simulink model "radio"  (R2023a)
settings: Solver=VariableStepAuto  StartTime=0.0  StopTime=10.0  RelTol=1e-3
libraries: dspvision x2, simulink x1, commanabbnd3 x1, zedboardfmc234_lib x1
settings Model: Creator=Lenovo  LastModifiedBy=Lenovo

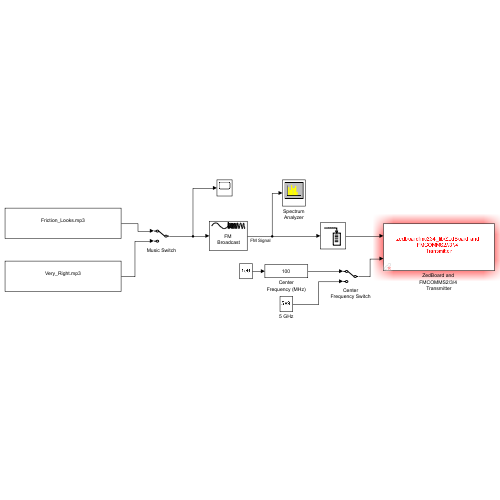
[thumbnail: Simulink's stored preview of the top-level diagram]
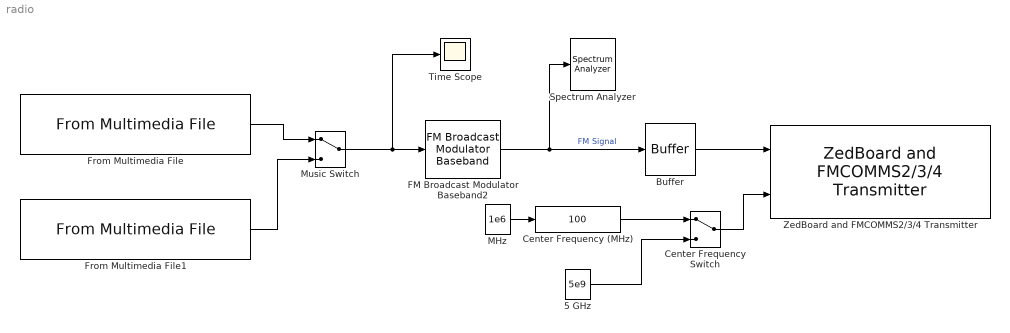
== system radio ==
  5 GHz : Constant  Value=5e9  VectorParams1D=off  SampleTime=192000/960000  FramePeriod=-1
  Buffer : Buffer  N=192000  OutputFrames=off
  Center Frequency (MHz) : simulink/Math Operations/Slider Gain  gain=100  low=98  high=102
  Center Frequency Switch : ManualSwitch
  FM Broadcast Modulator Baseband2 : commanabbnd3/FM Broadcast Modulator Baseband  SampleRate=960000  FrequencyDeviation=75000  FilterTimeConstant=7.5e-5  AudioSampleRate=48000  Stereo=on  RBDS=off  RBDSSamplesPerSymbol=10  SimulateUsing=Code generation
  From Multimedia File : dspvision/From Multimedia File  inputFilename=D:\LO_SHIH_AN\SDR\Matlab_object\SDR_FM_Radio\no_copyright_music\Friction_Looks.mp3  readRange=[1 Inf]  loop=on  numPlays=10  outputStreams=Audio only  videoDataType=single  audioDataType=double  inheritSampleTime=on  userDefinedSampleTime=1/4410  noAudioOutput=off  isIntensityVideo=off  fourcc=RGB  colorVideoFormat=Separate color signals  outputEOF=off  dataOrg=Column-major  audioFrameSize=48000  computeAudioFrameSize=off  outSamplingMode=Sample based
  From Multimedia File1 : dspvision/From Multimedia File  inputFilename=D:\LO_SHIH_AN\SDR\Matlab_object\SDR_FM_Radio\no_copyright_music\Very_Right.mp3  readRange=[1 Inf]  loop=on  numPlays=10  outputStreams=Audio only  videoDataType=single  audioDataType=double  inheritSampleTime=on  userDefinedSampleTime=1/4800  noAudioOutput=off  isIntensityVideo=off  fourcc=RGB  colorVideoFormat=Separate color signals  outputEOF=off  dataOrg=Column-major  audioFrameSize=48000  computeAudioFrameSize=off  outSamplingMode=Sample based
  MHz : Constant  Value=1e6  VectorParams1D=off  SampleTime=192000/960000  FramePeriod=-1
  Music Switch : ManualSwitch
  Spectrum Analyzer : SpectrumAnalyzer  WindowPosition=[1212 180 483 666]  ScopeFrameLocation=window  ViewType=Spectrum and spectrogram  Method=Welch  SampleRate=960000  Span=27930  StartFrequency=-13965  StopFrequency=13965  AveragingMethod=Running  YLimits=[-159.00256673081184999,35.803452450867595758]  ColorLimits=[-90.984095857497905513,17.091530854464384248]  ShowLegend=on  DefaultConfigurationName=spbscopes.SpectrumAnalyzerBlockCfg
  Time Scope : Scope
  ZedBoard and FMCOMMS2/3/4 Transmitter : zedboardfmc234_lib/ZedBoard and  FMCOMMS2//3//4  Transmitter  IPAddress=192.168.3.2  CenterFrequencySource=Input port  CenterFrequency=2400000000  GainSource=Dialog  Gain=0  ChannelMapping=1  BasebandSampleRate=960000  EnableBurstMode=off  NumFramesInBurst=20  DMATimeoutValue=1  EnableTxPrimingMode=on  blockMode=Normal  LostSamplesOutputPort=off  OverflowOutputPort=off  SimulateUsing=Code generation  DataSourceSelect=Host  DDSFrequency=[ 1000000, 1000000; 1000000, 1000000 ]  DDSPhase=[ 0, 0; 0, 0 ]  DDSScale=[ 250000, 250000; 250000, 250000 ]  BypassUserLogic=off  ShowAdvancedProperties=on  ShowInternalProperties=off  subDeviceList=zynqTransmitter  sdrExecutionMode=HW  dataUDPPort=-1  ctrlUDPPort=-1  FIRCoefficientSize=[ 128; 128 ]  FIRCoefficients=[ 111, -87, 147, -127, -18, -286, -312, -555, -601, -722, -642, -555, -303, -66, 221, 393, 488, 403, 219, -74, -343, -550, -582, -450, -146, 221, 569, 759, 735, 463, 20, -487, -885, -1048, -883, -418, 243, 897, 1340, 1394, 1002, 228, -715, -1549, -1980, -1819, -1028, 217, 1583, 2635, 2980, 2377, 853, -1275, -3435, -4926, -5080, -3454, 40, 5065, 10903, 16581, 21085, 23573, 23573, 21085, 16581, 10903, 5065, 40, -3454, -5080, -4926, -3435, -1275, 853, 2377, 2980, 2635, 1583, 217, -1028, -1819, -1980, -1549, -715, 228, 1002, 1394, 1340, 897, 243, -418, -883, -1048, -885, -487, 20, 463, 735, 759, 569, 221, -146, -450, -582, -550, -343, -74, 219, 403, 488, 393, 221, -66, -303, -555, -642, -722, -601, -555, -312, -286, -18, -127, 147, -87, 111; 382, -200, 711, -41, 645, 36, 346, -194, -119, -543, -472, -646, -404, -312, 45, 197, 413, 346, 241, -93, -373, -680, -755, -689, -356, 51, 515, 795, 870, 609, 136, -488, -1009, -1303, -1191, -712, 69, 885, 1516, 1692, 1336, 468, -662, -1740, -2378, -2329, -1494, -55, 1620, 2995, 3584, 3045, 1368, -1121, -3755, -5708, -6156, -4542, -710, 4969, 11669, 18243, 23486, 26391, 26391, 23486, 18243, 11669, 4969, -710, -4542, -6156, -5708, -3755, -1121, 1368, 3045, 3584, 2995, 1620, -55, -1494, -2329, -2378, -1740, -662, 468, 1336, 1692, 1516, 885, 69, -712, -1191, -1303, -1009, -488, 136, 609, 870, 795, 515, 51, -356, -689, -755, -680, -373, -93, 241, 346, 413, 197, 45, -312, -404, -646, -472, -543, -119, -194, 346, 36, 645, -41, 711, -200, 382 ]  FIRGain=[ 0; -12 ]  FIRDecimInterpFactor=[ 4; 4 ]  AnalogFilterCutoff=[ 2560000; 2560000 ]  FilterPathRates=[ 737280000, 184320000, 61440000, 30720000, 15360000, 3840000; 737280000, 184320000, 61440000, 30720000, 15360000, 3840000 ]  FilterDesignTypeForTx=DefaultFilter  FilterDesignTypeForRx=DefaultFilterFromOther
  wires:
  From Multimedia File/1 -> Music Switch/1
  From Multimedia File1/1 -> Music Switch/2
  FM Broadcast Modulator Baseband2/1 -> Buffer/1, Spectrum Analyzer/1  "FM Signal"
  Music Switch/1 -> Time Scope/1, FM Broadcast Modulator Baseband2/1
  5 GHz/1 -> Center Frequency Switch/2
  Center Frequency (MHz)/1 -> Center Frequency Switch/1
  Center Frequency Switch/1 -> ZedBoard and FMCOMMS2/3/4 Transmitter/2
  MHz/1 -> Center Frequency (MHz)/1
  Buffer/1 -> ZedBoard and FMCOMMS2/3/4 Transmitter/1
